simulink model "continuous_drone"  (R2021b)
settings: Solver=VariableStepAuto  StartTime=0.0  StopTime=10.0  RelTol=1e-3
values from neighbouring files (symbols this model uses):
  G_1 = [ mot_eff,mot_eff,mot_eff,mot_eff;0,-12.8,0,12.8;2.7,0,-2.7,0;-0.115,0.115,-0.115,0.115]./conv    [Model_Parameters.m]    (also in wls_test.m)
  G_2 = [0,0,0,0;0,0,0,0;0,0,0,0;-0.06,0.06,-0.06,0.06]./conv    [Model_Parameters.m]    (also in wls_test.m)
  motor_f = 18    [Model_Parameters.m]
libraries: simulink x1
settings Model: Creator=tomasodeponti  LastModifiedBy=tomasodeponti

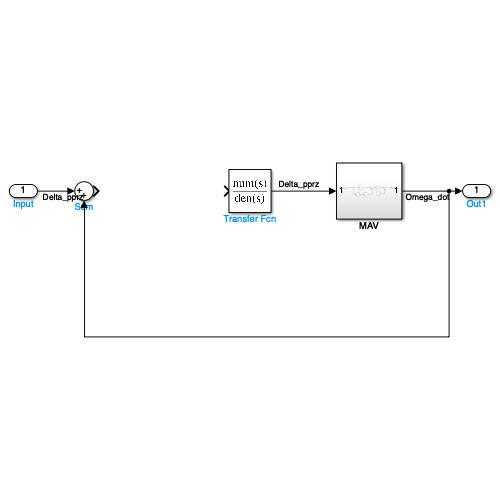
[thumbnail: Simulink's stored preview of the top-level diagram]
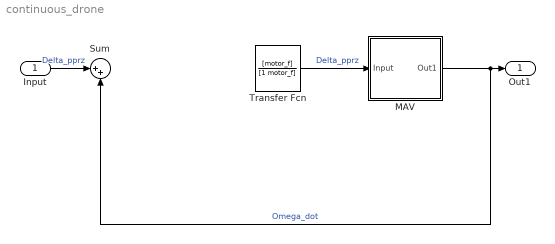
== system continuous_drone ==
  Input : Inport
  MAV : Subsystem
  Sum : Sum  Inputs=|++
  Transfer Fcn : TransferFcn  Numerator=[motor_f]  Denominator=[1 motor_f]
  Out1 : Outport  PortDimensions=3
  wires:
  Transfer Fcn/1 -> MAV/1(Input)  "Delta_pprz"
  MAV/1(Out1) -> Sum/2, Out1/1  "Omega_dot"
  Input/1 -> Sum/1  "Delta_pprz"

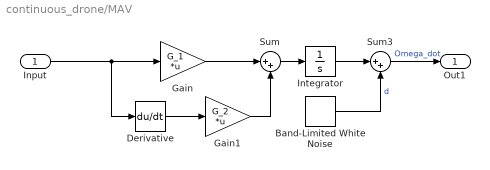
== system continuous_drone/MAV ==
  Input : Inport
  Band-Limited White Noise : simulink/Sources/Band-Limited White Noise  Cov=[0.1]  Ts=0.1  seed=[23341]
  Derivative : Derivative
  Gain : Gain  Gain=G_1  Multiplication=Matrix(K*u)
  Gain1 : Gain  Gain=G_2  Multiplication=Matrix(K*u)
  Integrator : Integrator
  Sum : Sum  Inputs=|++
  Sum3 : Sum  Inputs=|++
  Out1 : Outport  PortDimensions=3
  wires:
  Gain1/1 -> Sum/2
  Gain/1 -> Sum/1
  Input/1 -> Derivative/1, Gain/1
  Sum/1 -> Integrator/1
  Derivative/1 -> Gain1/1
  Band-Limited White Noise/1 -> Sum3/2  "d"
  Sum3/1 -> Out1/1  "Omega_dot"
  Integrator/1 -> Sum3/1
